simulink model "lab3"  (R2022a)
settings: Solver=VariableStepAuto  StartTime=0.0  StopTime=10.0  RelTol=1e-3
settings Model: Creator=1612918  LastModifiedBy=User
settings DebuggingCC: UnconnectedInputMsg=warning  UnconnectedOutputMsg=warning  UnconnectedLineMsg=warning
settings RTWCC: DLArmComputeVersion=19.05

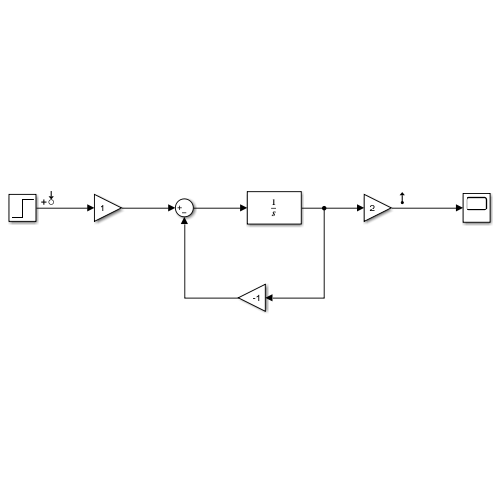
[thumbnail: Simulink's stored preview of the top-level diagram]
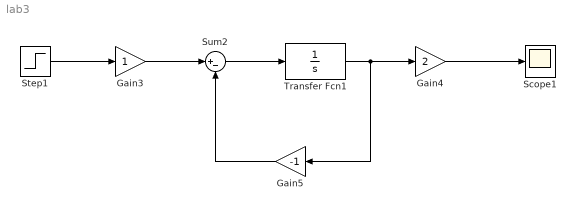
== system lab3 ==
  Gain3 : Gain
  Gain4 : Gain  Gain=2
  Gain5 : Gain  Gain=-1
  Scope1 : Scope
  Step1 : Step  SampleTime=0
  Sum2 : Sum  Inputs=|+-
  Transfer Fcn1 : TransferFcn  Denominator=[1 0]
  wires:
  Gain3/1 -> Sum2/1
  Transfer Fcn1/1 -> Gain5/1, Gain4/1
  Gain4/1 -> Scope1/1
  Sum2/1 -> Transfer Fcn1/1
  Gain5/1 -> Sum2/2
  Step1/1 -> Gain3/1
